simulink model "DriftingController_Stabilization"  (R2017a)
settings: Solver=FixedStepAuto  StartTime=0.0  StopTime=inf  FixedStep=0.01  RelTol=1e-3
InitFcn:
  | DriftingController_Stabilization_CallbackFunction
values from neighbouring files (symbols this model uses):
  delta_eqpoint = -10*pi/180    (= -0.174532925199)    [DriftingController_Stabilization_CallbackFunction.m]
  delta_max = 35*pi/180    (= 0.610865238198)    [DriftingController_Stabilization_CallbackFunction.m]
  delta_min = -delta_max    (= -0.610865238198)    [DriftingController_Stabilization_CallbackFunction.m]
  Fdrag = 2    [DriftingController_Stabilization_CallbackFunction.m]
  FilterDTF = c2d(F,Ts,'tustin')    [DriftingController_Stabilization_CallbackFunction.m]
  Fxr_eqpoint = 1.25488    [DriftingController_Stabilization_CallbackFunction.m]
  Imax = 10    [DriftingController_Stabilization_CallbackFunction.m]
  K = [-0.1667   -0.2873    0.6444 ... (first row only)    [DriftingController_Stabilization_CallbackFunction.m]
  Kt = 1/340.34    (= 0.00293823823236)    [DriftingController_Stabilization_CallbackFunction.m]
  r_eqpoint = 1.24259    [DriftingController_Stabilization_CallbackFunction.m]
  Rw = 0.049    [DriftingController_Stabilization_CallbackFunction.m]
  tau = 0.1159    [DriftingController_Stabilization_CallbackFunction.m]
  Vx_eqpoint = 1.5    [DriftingController_Stabilization_CallbackFunction.m]
  Vy_eqpoint = -0.6100    (= -0.61)    [DriftingController_Stabilization_CallbackFunction.m]
undefined symbols (not defined in the file or in its folder): SpeedRef, State, SteerRef
libraries: robotlib x5
settings Model: Creator=bascetta  LastModifiedBy=marco
settings OptimizationCC: PassReuseOutputArgsAs=Individual arguments  MaxStackSize=64
settings DebuggingCC: ParameterTunabilityLossMsg=error
settings HardwareCC: ProdBitPerPointer=32  ProdBitPerSizeT=32  ProdBitPerPtrDiffT=32  ProdLargestAtomicFloat=None  ProdIntDivRoundTo=Undefined  ProdEndianess=Unspecified  ProdWordSize=32  ProdHWDeviceType=Generic->Unspecified (assume 32-bit Generic)
settings SFSimCC: MATLABDynamicMemAlloc=off
settings RTWCC: SystemTargetFile=ert.tlc  HardwareBoard=Robot Operating System (ROS)  TLCOptions="-aInlineSetEventsForThisBaseRateFcn=TLC_FALSE -aSuppressMultiTaskScheduler=TLC_FALSE  -aRateBasedStepFcn=0"  TemplateMakefile=ert_default_tmf  Description=Embedded Coder  GenerateReport=on  Toolchain=Catkin  IncludeHyperlinkInReport=on  LaunchReport=on  TargetLang=C++  GenerateTraceInfo=on  GenerateTraceReport=on  GenerateTraceReportSl=on  GenerateTraceReportSf=on  GenerateTraceReportEml=on
settings CodeAppCC: ForceParamTrailComments=on  IgnoreCustomStorageClasses=off  OperatorAnnotations=on  SimulinkDataObjDesc=on  SFDataObjDesc=on  MATLABFcnDesc=on  InsertBlockDesc=on  MATLABSourceComments=on
settings ERTTargetCC: SupportContinuousTime=on
settings ConfigComp: CovScope=ReferencedModels  CovIncludeTopModel=off

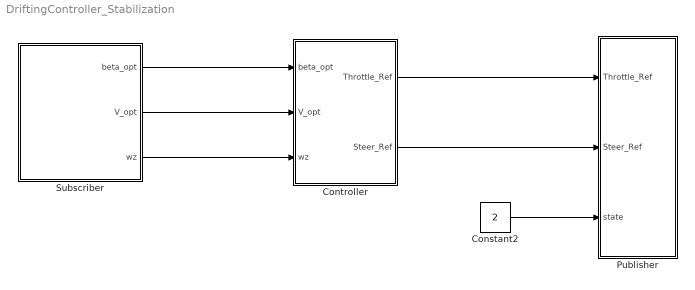
== system DriftingController_Stabilization ==
  Constant2 : Constant  Value=2  OutDataTypeStr=uint8
  Controller : Subsystem
  Publisher : Subsystem
  "Subscriber " : Subsystem
  wires:
  Constant2/1 -> Publisher/3(state)
  "Subscriber "/1(beta_opt) -> Controller/1(beta_opt)
  Controller/1(Throttle_Ref) -> Publisher/1(Throttle_Ref)
  Controller/2(Steer_Ref) -> Publisher/2(Steer_Ref)
  "Subscriber "/3(wz) -> Controller/3(wz)
  "Subscriber "/2(V_opt) -> Controller/2(V_opt)

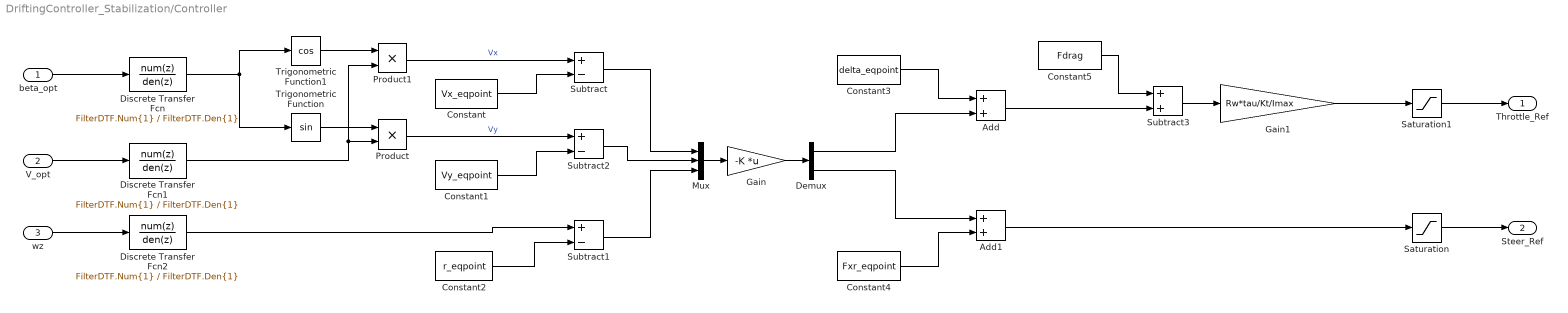
== system DriftingController_Stabilization/Controller ==
  beta_opt : Inport
  V_opt : Inport  Port=2
  wz : Inport  Port=3
  Add : Sum
  Add1 : Sum
  Constant : Constant  Value=Vx_eqpoint
  Constant1 : Constant  Value=Vy_eqpoint
  Constant2 : Constant  Value=r_eqpoint
  Constant3 : Constant  Value=delta_eqpoint
  Constant4 : Constant  Value=Fxr_eqpoint
  Constant5 : Constant  Value=Fdrag
  Demux : Demux  Outputs=2
  Discrete Transfer Fcn : DiscreteTransferFcn  Numerator=FilterDTF.Num{1}  Denominator=FilterDTF.Den{1}
  Discrete Transfer Fcn1 : DiscreteTransferFcn  Numerator=FilterDTF.Num{1}  Denominator=FilterDTF.Den{1}
  Discrete Transfer Fcn2 : DiscreteTransferFcn  Numerator=FilterDTF.Num{1}  Denominator=FilterDTF.Den{1}
  Gain : Gain  Gain=-K  Multiplication=Matrix(K*u)
  Gain1 : Gain  Gain=Rw*tau/Kt/Imax
  Mux : Mux  Inputs=3
  Product : Product
  Product1 : Product
  Saturation : Saturate  UpperLimit=delta_max  LowerLimit=delta_min
  Saturation1 : Saturate  UpperLimit=1  LowerLimit=-1
  Subtract : Sum  Inputs=+-
  Subtract1 : Sum  Inputs=+-
  Subtract2 : Sum  Inputs=+-
  Subtract3 : Sum
  Trigonometric Function : Trigonometry
  Trigonometric Function1 : Trigonometry  Operator=cos
  Throttle_Ref : Outport
  Steer_Ref : Outport  Port=2
  wires:
  beta_opt/1 -> Discrete Transfer Fcn/1
  V_opt/1 -> Discrete Transfer Fcn1/1
  wz/1 -> Discrete Transfer Fcn2/1
  Discrete Transfer Fcn/1 -> Trigonometric Function/1, Trigonometric Function1/1
  Trigonometric Function1/1 -> Product1/1
  Trigonometric Function/1 -> Product/1
  Discrete Transfer Fcn1/1 -> Product/2, Product1/2
  Mux/1 -> Gain/1
  Product1/1 -> Subtract/1  "Vx"
  Product/1 -> Subtract2/1  "Vy"
  Discrete Transfer Fcn2/1 -> Subtract1/1
  Constant/1 -> Subtract/2
  Constant1/1 -> Subtract2/2
  Constant2/1 -> Subtract1/2
  Gain/1 -> Demux/1
  Demux/2 -> Add1/1
  Add1/1 -> Saturation/1
  Demux/1 -> Add/2
  Constant3/1 -> Add/1
  Constant4/1 -> Add1/2
  Subtract/1 -> Mux/1
  Subtract2/1 -> Mux/2
  Subtract1/1 -> Mux/3
  Add/1 -> Subtract3/2
  Constant5/1 -> Subtract3/1
  Subtract3/1 -> Gain1/1
  Gain1/1 -> Saturation1/1
  Saturation/1 -> Steer_Ref/1
  Saturation1/1 -> Throttle_Ref/1

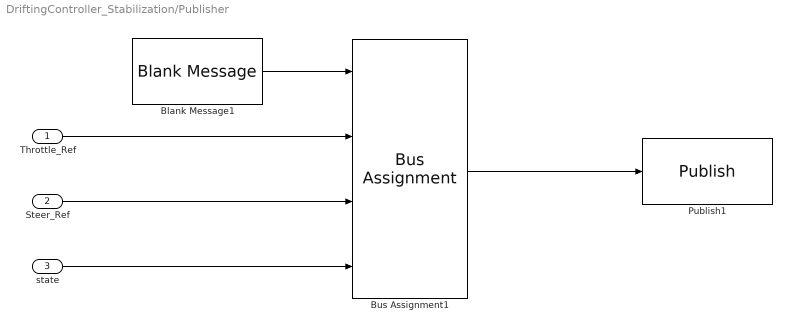
== system DriftingController_Stabilization/Publisher ==
  Throttle_Ref : Inport
  Steer_Ref : Inport  Port=2
  state : Inport  Port=3
  Blank Message1 : robotlib/Blank Message  SourceLibraryInfo=This block requires Robotics System Toolbox  messageType=car_msgs/car_cmd  SampleTime=inf
      settings: SourceProductBaseCode=RO
  Bus Assignment1 : BusAssignment  AssignedSignals=SpeedRef,SteerRef,State
  Publish1 : robotlib/Publish  SourceLibraryInfo=This block requires Robotics System Toolbox  topicSource=Specify your own  topic=/controller_cmd  messageType=car_msgs/car_cmd  messageQueueLength=1
      settings: SourceProductBaseCode=RO
  wires:
  Blank Message1/1 -> Bus Assignment1/1
  Bus Assignment1/1 -> Publish1/1
  Throttle_Ref/1 -> Bus Assignment1/2
  Steer_Ref/1 -> Bus Assignment1/3
  state/1 -> Bus Assignment1/4

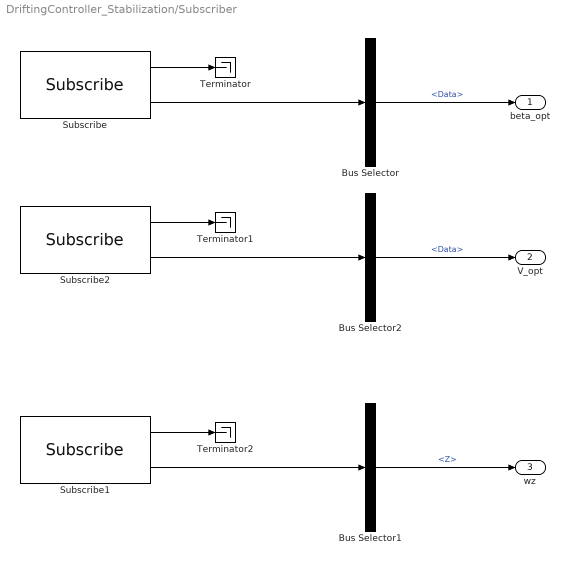
== system DriftingController_Stabilization/Subscriber  ==
  Bus Selector : BusSelector  OutputSignals=Data
  Bus Selector1 : BusSelector  OutputSignals=AngularVelocity.Z
  Bus Selector2 : BusSelector  OutputSignals=Data
  Subscribe : robotlib/Subscribe  SourceLibraryInfo=This block requires Robotics System Toolbox  topicSource=Select from ROS network  topic=/state_estimator_opt_beta  messageType=std_msgs/Float64  sampleTime=-1  messageQueueLength=1
      settings: SourceProductBaseCode=RO
  Subscribe1 : robotlib/Subscribe  SourceLibraryInfo=This block requires Robotics System Toolbox  topicSource=Select from ROS network  topic=/imu/data  messageType=sensor_msgs/Imu  sampleTime=-1  messageQueueLength=1
      settings: SourceProductBaseCode=RO
  Subscribe2 : robotlib/Subscribe  SourceLibraryInfo=This block requires Robotics System Toolbox  topicSource=Select from ROS network  topic=/state_estimator_opt_V  messageType=std_msgs/Float64  sampleTime=-1  messageQueueLength=1
      settings: SourceProductBaseCode=RO
  Terminator : Terminator
  Terminator1 : Terminator
  Terminator2 : Terminator
  beta_opt : Outport
  V_opt : Outport  Port=2
  wz : Outport  Port=3
  wires:
  Subscribe/2 -> Bus Selector/1
  Subscribe2/2 -> Bus Selector2/1
  Bus Selector/1 -> beta_opt/1  "<Data>"
  Bus Selector2/1 -> V_opt/1  "<Data>"
  Subscribe/1 -> Terminator/1
  Subscribe2/1 -> Terminator1/1
  Subscribe1/1 -> Terminator2/1
  Subscribe1/2 -> Bus Selector1/1
  Bus Selector1/1 -> wz/1  "<Z>"
